simulink model "Cascade_Control_CRP_Simulink"  (R2021a)
settings: Solver=VariableStepAuto  StartTime=0.0  StopTime=20  MaxStep=0.001  RelTol=1e-3
undefined symbols (not defined in the file): ang, c, Cf, Den_D_d, Den_m, g, kp, m, Num_D_d, Num_m, physical_constraint, sp, static_friction, Tm, Ts, w0, wsp
libraries: simulink x2, simulink_extras x1
settings Model: Creator=xavie  LastModifiedBy=Administrateur
settings SolverCC: AlgebraicLoopSolver=TrustRegion
settings DebuggingCC: SFMachineParentedDataDiag=warning

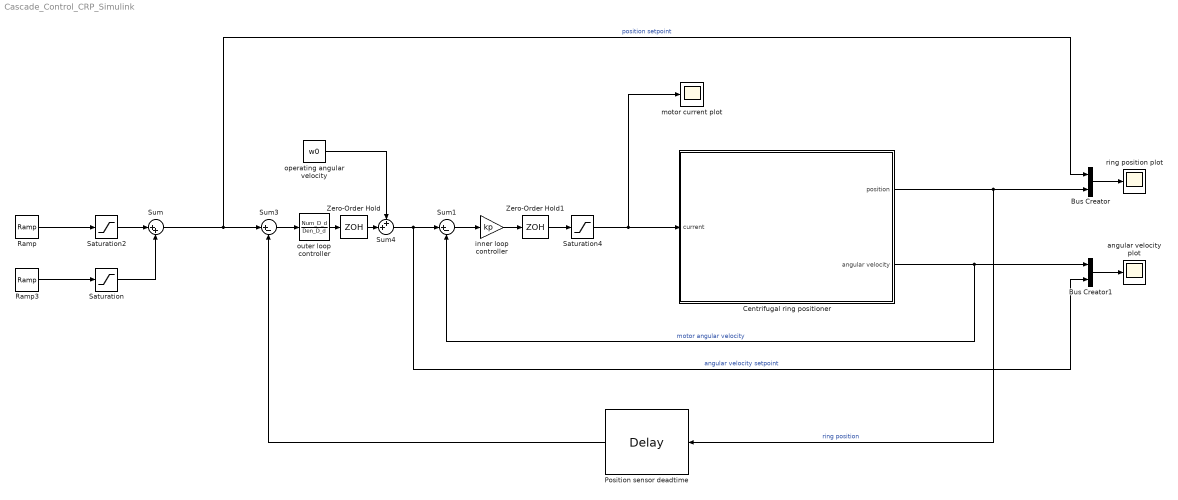
== system Cascade_Control_CRP_Simulink ==
  Bus Creator : BusCreator  Inputs=2
  Bus Creator1 : BusCreator  Inputs=2
  Centrifugal ring positioner : Subsystem
      mask Display: image('C:\Users\Administrateur\OneDrive - Université Libre de Bruxelles\Documents\Xavier\Cours Polytech\Master Thesis\Design\Assemblage_SW_4.PNG'); % Use "Edit Image" on toolstrip to change.
  "Position sensor deadtime " : TransportDelay  DelayTime=Tm  InitialOutput=sp
      mask Display: image('C:\Users\Administrateur\OneDrive - Université Libre de Bruxelles\Documents\Xavier\Cours Polytech\Master Thesis\Design\Sharp_GP2Y.PNG'); % Use "Edit Image" on toolstrip to change.
  Ramp : simulink/Sources/Ramp  slope=0.016  start=0  InitialOutput=sp  VectorParams1D=off
  Ramp3 : simulink/Sources/Ramp  slope=-0.008  start=10  InitialOutput=0
  Saturation : Saturate  UpperLimit=11  LowerLimit=-0.04
  Saturation2 : Saturate  UpperLimit=sp+0.08  LowerLimit=0
  Saturation4 : Saturate  UpperLimit=0.652  LowerLimit=-0.652
  Sum : Sum  Inputs=|++
  Sum1 : Sum  Inputs=|+-
  Sum3 : Sum  Inputs=|+-
  Sum4 : Sum  Inputs=++|
  Zero-Order Hold : ZeroOrderHold  SampleTime=Ts/2
  Zero-Order Hold1 : ZeroOrderHold  SampleTime=Ts/2
  angular velocity plot : Scope
  inner loop controller : Gain  Gain=kp
  motor current plot : Scope
  operating angular velocity : Constant  Value=w0
  outer loop controller : DiscreteTransferFcn  Numerator=Num_D_d  Denominator=Den_D_d  SampleTime=Ts
  ring position plot : Scope
  wires:
  "Position sensor deadtime "/1 -> Sum3/2
  Saturation4/1 -> motor current plot/1, Centrifugal ring positioner/1("current ")
  Sum/1 -> Bus Creator/1, Sum3/1  "position setpoint"
  Sum1/1 -> inner loop controller/1
  Centrifugal ring positioner/1(position) -> Bus Creator/2, "Position sensor deadtime "/1  "ring position"
  operating angular velocity/1 -> Sum4/1
  outer loop controller/1 -> Zero-Order Hold/1
  Sum4/1 -> Sum1/1, Bus Creator1/2  "angular velocity setpoint"
  inner loop controller/1 -> Zero-Order Hold1/1
  Sum3/1 -> outer loop controller/1
  Zero-Order Hold1/1 -> Saturation4/1
  Ramp3/1 -> Saturation/1
  Saturation2/1 -> Sum/1
  Saturation/1 -> Sum/2
  Ramp/1 -> Saturation2/1
  Zero-Order Hold/1 -> Sum4/2
  Bus Creator/1 -> ring position plot/1
  Bus Creator1/1 -> angular velocity plot/1
  Centrifugal ring positioner/2(angular velocity) -> Sum1/2, Bus Creator1/1  "motor angular velocity"

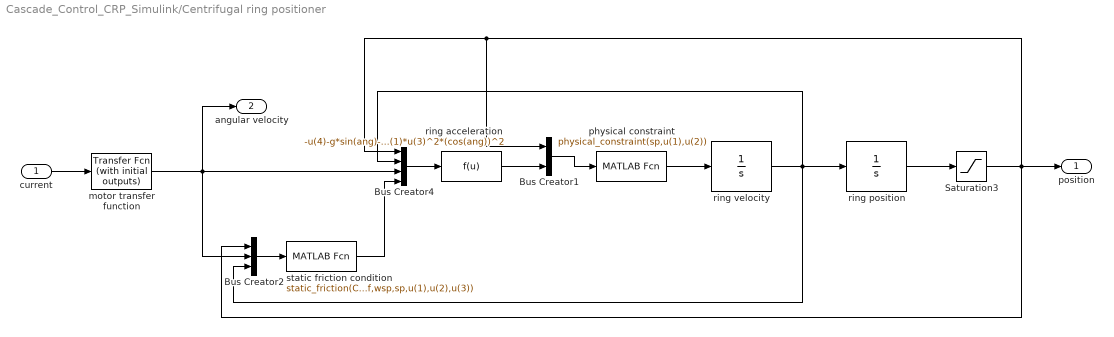
== system Cascade_Control_CRP_Simulink/Centrifugal ring positioner ==
  "current " : Inport
  Bus Creator1 : BusCreator  Inputs=2
  Bus Creator2 : BusCreator  Inputs=3
  Bus Creator4 : BusCreator  Inputs=4
  Saturation3 : Saturate  UpperLimit=0.206  LowerLimit=-55
  motor transfer function : simulink_extras/Additional Linear/Transfer Fcn (with initial outputs)  N=Num_m  D=Den_m  Y0=wsp  U0=0
  physical constraint : MATLABFcn  MATLABFcn=physical_constraint(sp,u(1),u(2))  OutputDimensions=1
  ring acceleration : Fcn  Expr=-u(4)-g*sin(ang)-c*u(2)/m+u(1)*u(3)^2*(cos(ang))^2
  ring position : Integrator  InitialCondition=sp
  ring velocity : Integrator
  static friction condition : MATLABFcn  MATLABFcn=static_friction(Cf,wsp,sp,u(1),u(2),u(3))  OutputDimensions=1
  position : Outport
  angular velocity : Outport  Port=2
  wires:
  "current "/1 -> motor transfer function/1
  motor transfer function/1 -> angular velocity/1, Bus Creator2/2, Bus Creator4/3
  Bus Creator4/1 -> ring acceleration/1
  Bus Creator1/1 -> physical constraint/1
  ring velocity/1 -> Bus Creator2/3, ring position/1, Bus Creator4/2
  Saturation3/1 -> Bus Creator1/1, Bus Creator4/1, position/1, Bus Creator2/1
  physical constraint/1 -> ring velocity/1
  Bus Creator2/1 -> static friction condition/1
  static friction condition/1 -> Bus Creator4/4
  ring position/1 -> Saturation3/1
  ring acceleration/1 -> Bus Creator1/2
